simulink model "FSKMethod2"  (R2019b)
settings: Solver=VariableStepAuto  StartTime=0.0  StopTime=1  RelTol=1e-3
settings Model: Creator=z3454314  LastModifiedBy=z3454314

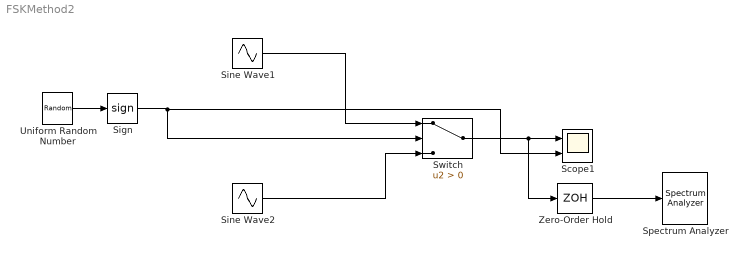
== system FSKMethod2 ==
  Scope1 : Scope  NumInputPorts=2
  Sign : Signum
  Sine Wave1 : Sin  Frequency=2000*2*pi  SampleTime=0
  Sine Wave2 : Sin  Frequency=8000*2*pi  SampleTime=0
  Spectrum Analyzer : SpectrumAnalyzer
  Switch : Switch  Criteria=u2 > Threshold
  Uniform Random Number : UniformRandomNumber  SampleTime=1/280
  Zero-Order Hold : ZeroOrderHold  SampleTime=1/44100
  wires:
  Uniform Random Number/1 -> Sign/1
  Sine Wave2/1 -> Switch/3
  Sine Wave1/1 -> Switch/1
  Switch/1 -> Zero-Order Hold/1, Scope1/1
  Zero-Order Hold/1 -> Spectrum Analyzer/1
  Sign/1 -> Switch/2, Scope1/2
